simulink model "HD2_Driver_PY_v3"  (R2018a)
settings: Solver=ode1  StartTime=0.0  StopTime=inf  FixedStep=0.001  RelTol=1e-3  EnableMultiTasking=on
InitFcn:
  | % Assign block mask parameter to variable in base workspace
  | mdlPrefix_hd2_py = 'HD2_PY_';
  | mdlName_hd2_py = 'HD2_Driver_PY_v3';
  | blkName_hd2_py = 'HD2_Parameters';
  | blkRef_hd2_py = strcat(mdlName_hd2_py, '/', blkName_hd2_py);
  | 
  | % Extract list of parameters defined in the "HD2 Parameter" subsystem block
  | dialogParams_hd2_py = get_param( blkRef_hd2_py,'DialogParameters');
  | dialogParamsNames_hd2_py = fieldnames(dialogParams_hd2_py);
  | 
  | % Assign each parameter to a variable with mdlPrefix<param_name> formatted name
  | for idx = 1:numel(dialogParamsNames_hd2_py)
  |     paramVal = eval( get_param( blkRef_hd2_py, dialogParamsNames_hd2_py{idx} ) );
  |     assignin( 'base', strcat(mdlPrefix_hd2_py,dialogParamsNames_hd2_py{idx}), paramVal);
  | end
  | 
model workspace (MAT data in the model file):
  ErrTol = Simulink.Parameter
  ErrTol.Value = 0.0001
  ErrTol.DataType = 'auto'
  ErrTol.Dimensions = [1 1]
undefined symbols (not defined in the file): HD2_PY_CalibHome, HD2_PY_HandleLength, HD2_PY_HandleOffset, HD2_PY_HandleTol, HD2_PY_LinkLengths, HD2_PY_MotorAmpGains, HD2_PY_MotorAmpLimits, HD2_PY_QDirs, HD2_PY_QEnc, HD2_PY_QGains, HD2_PY_QKv, HIL, qc_get_step_size
libraries: quarc_library x30, simulink x10, simulink_extras x6
(part 1 of 2)
settings Model: SimulationMode=external  ExtModeTrigDuration=10000  Creator=glai  LastModifiedBy=mrushton
settings SolverCC: PositivePriorityOrder=on
settings RTWCC: Description=QUARC Win64 Target Using Toolchain  SystemTargetFile=quarc_win64.tlc  TemplateMakefile=quarc_default_tmf  Toolchain=QUARC win64 | nmake (64-bit Windows)  BuildConfiguration=Faster Runs
settings CodeAppCC: StateflowObjectComments=on
settings STFCustomTargetCC: TargetLangStandard=C99 (ISO)  ConcurrentExecutionCompliant=on  UseToolchainInfoCompliant=on  SystemTargetFile=quarc_win64.tlc
settings GRTTargetCC: ParMdlRefBuildCompliant=off  CompOptLevelCompliant=off  CombineOutputUpdateFcns=off  MatFileLogging=off  CPPClassGenCompliant=off  GRTInterface=on  ExtMode=on  ExtModeMexFile=quarc_comm  ExtModeMexArgs='-w -d %d -uri %u -URI_SHMEM shmem://HD2_DRIVER_PY:0','tcpip://localhost:17001'
settings ConfigComp: CovMetricSettings=dswe

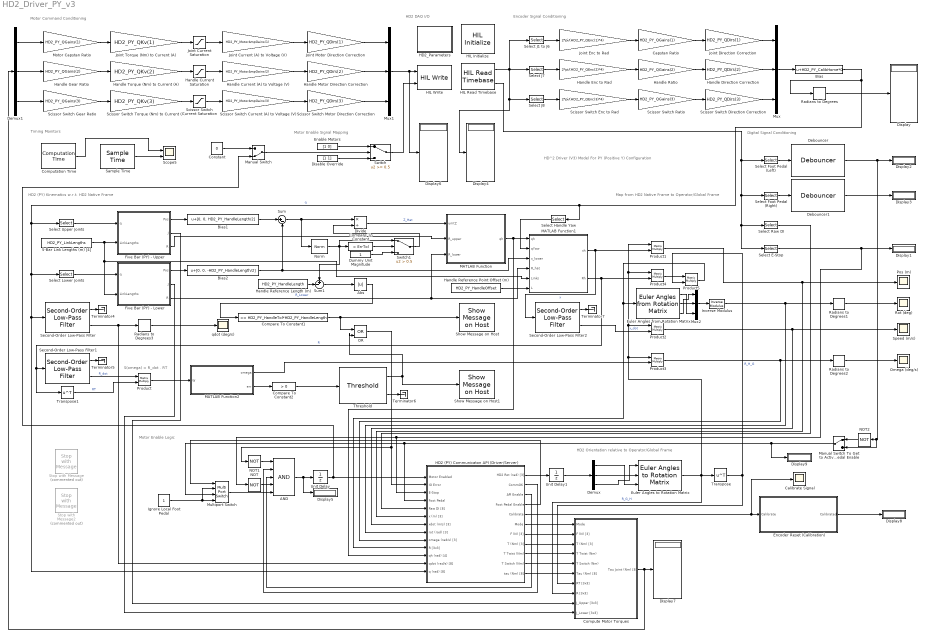
== system HD2_Driver_PY_v3 ==
  note: Motor Enable Logic
  note: Timing Monitors
  note: Map from HD2 Native Frame to Operator/Global Frame
  note: S(omega) = R_dot . RT
  note: HD2 (PY) Kinematics w.r.t. HD2 Native Frame
  note: HD2 Orientation relative to Operator/Global Frame
  note: Motor Enable Signal Mapping
  note: Motor Command Conditioning
  note: Digital Signal Conditioning
  note: Encoder Signal Conditioning
  note: HD2 DAQ I/O
  note: HD^2 Driver (V3) Model For PY (Positive Y) Configuration
  5-Bar Link Lengths (m) [4] : Constant  Value=HD2_PY_LinkLengths
  AND : Logic  Inputs=5  IconShape=distinctive  AllPortsSameDT=off  OutDataTypeStr=boolean
  Abs : Abs
  Bias : Bias  Bias=HD2_PY_CalibHome*0
  Bias1 : Bias  Bias=[0, 0, HD2_PY_HandleLength/2]
  Bias2 : Bias  Bias=[0, 0, -HD2_PY_HandleLength/2]
  Calibrate Signal : Scope
  Capstan Ratio : Gain  Gain=HD2_PY_QGains(1)
  Compare To Constant : simulink/Logic and Bit Operations/Compare To Constant  relop=>  const=ErrTol  OutDataTypeStr=boolean
  Compare To Constant1 : simulink/Logic and Bit Operations/Compare To Constant  relop=>=  const=HD2_PY_HandleTol*HD2_PY_HandleLength  OutDataTypeStr=boolean
  Compare To Constant2 : simulink/Logic and Bit Operations/Compare To Constant  relop=>  const=0  OutDataTypeStr=boolean
  Computation Time : quarc_library/Sources/Time/Computation Time  sample_time=qc_get_step_size  use_model=on  use_cpu_time=off
  Compute Motor Torques : Subsystem
  Constant : Constant  Value=0
  Debouncer : quarc_library/Discontinuities/Debouncer  init_state=Off  param_src=Specify via dialog  threshold=0.5  rise_time=0.01  fall_time=0.01
      settings: SourceProductName=QUARC Targets
  Debouncer1 : quarc_library/Discontinuities/Debouncer  init_state=Off  param_src=Specify via dialog  threshold=0.5  rise_time=0.01  fall_time=0.01
      settings: SourceProductName=QUARC Targets
  Demux : Demux  Outputs=3
  Demux1 : Demux  Outputs=[6 1 1]
  Disable Override : Constant  Value=[1 1]
  Display{,1..9} (10 alike) : Display
      settings: Decimation=100
  Divide : Product  Inputs=*/
  Dummy Unit Magnitude : Constant
  Enable Motors : Constant  Value=[1 0]
  Encoder Reset (Calibration) : Subsystem
  Euler Angles from Rotation Matrix : quarc_library/Math Operations/Matrices/Euler Angles from Rotation Matrix  menu_order=Relative Z-Y-X
      settings: SourceProductName=QUARC Targets
  Euler Angles to Rotation Matrix : quarc_library/Math Operations/Matrices/Euler Angles to Rotation Matrix  menu_order=Relative Z-Y-X
      settings: SourceProductName=QUARC Targets
  Five Bar (PY) - Lower : MATLAB Function  TreatAsAtomicUnit=on
  Five Bar (PY) - Upper : MATLAB Function  TreatAsAtomicUnit=on
  HD2 (PY) Communicaton API (Driver/Server) : Subsystem
  HD2_Parameters : Subsystem  Priority=-100  TreatAsAtomicUnit=on  mask{CalibHome=[-2, -14.5, 106, -2, -14.5, 106.5, 0, 0 ] * pi/180, HandleLength=0.175, HandleTol=0.1, HandleOffset=0.175/2, LinkLengths=[0.115, 0.28, 0.28, 0.022], QEnc=[1000, 360, 512], QGains=[1/12, 1, 1], QDirs=[-1, -1, 1], QKv=[1/115e-3, 1/0.0058, 1/0.0058], MotorAmpGains=[2.41, 2, 2], MotorAmpLimits=[5, 0.6, 0.6]}
      mask prompts: CalibHome "Joint Angles at Holder Home (rad) [8] :"; HandleLength "Handle Length/Anchor Offset (m) :"; HandleTol "Handle Length Tolerance (%) :"; HandleOffset "EE Reference Offset from base (m) :"; LinkLengths "5-Bar Link Lengths (m) [4] :"; QEnc "Encoder Resolutions (lines per rev) [3] :"; QGains "Capstan Gains/Gear Ratio [3] :"; QDirs "Direction Correction [3] :"; QKv "Torque Constant Inverse (1/Kt) (A/Nm) [3] :"; MotorAmpGains "Amplifier Resolution (V/A) [3] :"; MotorAmpLimits "Amplifier Current Limits (A) [3] :"
      mask help:
      | HD2 Parameters - PY Configuration
      |
      | The joint outputs are organized as follows (re-mapped from the encoder channel ordering):
      |
      | J1: Top 5-Bar base joint (Encoder Channel 2)
      | J2: Top 5-Bar first joint (Encoder Channel 1)
      | J3: Top 5-Bar second joint (Encoder Channel 0)
      | J4: Bottom 5-Bar base joint (Encoder Channel 5)
      | J5: Bottom 5-Bar first joint (Encoder Channel 4)
      | J6: Bottom 5-Bar second joint (Encoder Channel 3)
      | J7: Handle (Twist) joint (Encoder Channel 6)
      | J8: Scissor Switch joint (Encoder Channel 7)
      |
      | For the Joint and Motor parameters, the first 6 joints have the same values and therefore the parameter values are specified as a vector of three elements with the first element applying to J1 to J6 while the remaining elements apply to J7 and J8.
      mask init:
      | % Assign block mask parameter to variable in base workspace
      | %mdlPrefix = 'HD2_PY_';
      | 
      | %assignin( 'base', strcat(mdlPrefix,'CalibHome'), CalibHome);
      | %assignin( 'base', strcat(mdlPrefix,'HandleLength'), HandleLength);
      | %assignin( 'base', strcat(mdlPrefix,'HandleTol'), HandleTol);
      | %assignin( 'base', strcat(mdlPrefix,'HandleOffset'), HandleOffset);
      | %assignin( 'base', strcat(mdlPrefix,'LinkLengths'), LinkLengths);
      | %assignin( 'base', strcat(mdlPrefix,'QEnc'), QEnc);
      | %assignin( 'base', strcat(mdlPrefix,'QGains'), QGains);
      | %assignin( 'base', strcat(mdlPrefix,'QDirs'), QDirs);
      | %assignin( 'base', strcat(mdlPrefix,'QKv'), QKv);
      | %assignin( 'base', strcat(mdlPrefix,'MotorAmpGains'), MotorAmpGains);
      | %assignin( 'base', strcat(mdlPrefix,'MotorAmpLimits'), MotorAmpLimits);
      mask DialogControl CalibGroupVar Prompt: Calibration Parameters
      mask DialogControl ParameterGroupVar Prompt: Handle and Link Parameters
      mask DialogControl JointParamGroupVar Prompt: Joint Parameters
      mask DialogControl MotorParamGroupVar Prompt: Motor Parameters
      mask Display: disp('HD2\nParameters\n(Double-Click\nto edit)');
  HIL Initialize : quarc_library/Data Acquisition/Generic/Configuration/HIL Initialize  Priority=-99  object_name=HIL-1  board_type=qpid_e  board_number=0  board_options=enc0_dir=0;enc0_filter=1;enc0_a=1;enc0_b=1;enc0_z=0;enc0_reload=0;enc1_dir=0;enc1_filter=1;enc1_a=1;enc1_b=1;enc1_z=0;enc1_reload=0;enc2_dir=0;enc2_filter=1;enc2_a=1;enc2_b=1;enc2_z=0;enc2_reload=0;enc3_dir=0;enc3_filter=1;enc3_a=1;enc3_b=1;enc3_z=0;enc3_reload=0;enc4_dir=0;enc4_filter=1;enc4_a=1;enc4_b=1;enc4_z=0;enc4_reload=0;enc5_dir=0;enc5_filter=1;enc5_a=1;enc5_b=1;enc5_z=0;enc5_reload=0;enc6_dir=0;enc6_filter=1;enc6_a=1;enc6_b=1;enc6_z=0;enc6_reload=0;enc7_dir=0;enc7_filter=1;enc7_a=1;enc7_b=1;enc7_z=0;enc7_reload=0;ext_int_polarity=0;fuse_polarity=0;convert_polarity=0;watchdog_polarity=0;ext_int_watchdog=0;fuse_watchdog=0;trig1_watchdog=0;watchdog_to_trig1=0;watchdog_to_trig2=0;counter_to_trig0=0;trigger_adcs=0;latch_on_adc=0;pwm_immediate=0  exclusive=off  active=off  hardware_clocks=[0:16]  clock_modes=[]  initial_clock_frequencies=[]  set_clock_params_at_start=off  set_clock_params_at_switch_in=off  set_clock_frequencies_at_start=off  set_clock_frequencies_at_switch_in=off  analog_input_channels=[0:7]  analog_input_configurations=0  analog_input_maximums=10  analog_input_minimums=-10  set_analog_input_params_at_start=off  set_analog_input_params_at_switch_in=off  analog_output_channels=[0:7]  analog_output_maximums=10  analog_output_minimums=-10  initial_analog_outputs=[0]  final_analog_outputs=[0]  watchdog_analog_outputs=0  set_analog_output_params_at_start=off  set_analog_output_params_at_switch_in=off  set_analog_outputs_at_start=on  set_analog_outputs_at_switch_in=off  set_analog_outputs_at_terminate=on  set_analog_outputs_at_switch_out=off  set_analog_outputs_on_watchdog=off  digital_input_channels=[0:1,11]  digital_output_channels=[9:10]  digital_output_configuration=[]  initial_digital_outputs=[1]  final_digital_outputs=[1]  watchdog_digital_outputs=[2]  set_digital_output_params_at_start=off  set_digital_output_params_at_switch_in=off  set_digital_outputs_at_start=on  set_digital_outputs_at_switch_in=off  set_digital_outputs_at_terminate=on  set_digital_outputs_at_switch_out=off  set_digital_outputs_on_watchdog=off  encoder_channels=[0:7]  quadrature=[4]  encoder_filter_frequency=40e6/1  initial_encoder_counts=[0]  set_encoder_params_at_start=off  set_encoder_params_at_switch_in=off  set_encoder_counts_at_start=off  set_encoder_counts_at_switch_in=off  pwm_channels=[0:7]  pwm_modes=0  pwm_frequency=40e6/4096  pwm_configuration=[0]  pwm_alignment=[0]  pwm_polarity=[1]  pwm_leading_deadband=[0]  pwm_trailing_deadband=[0]  initial_pwm_outputs=[0]  final_pwm_outputs=[0]  watchdog_pwm_outputs=[0]  set_pwm_params_at_start=on  set_pwm_params_at_switch_in=off  set_pwm_outputs_at_start=on  set_pwm_outputs_at_switch_in=off  set_pwm_outputs_at_terminate=on  set_pwm_outputs_at_switch_out=off  set_pwm_outputs_on_watchdog=off  other_output_channels=[]  initial_other_outputs=[]  final_other_outputs=[]  watchdog_other_outputs=[]  set_other_outputs_at_start=off  set_other_outputs_at_switch_in=off  set_other_outputs_at_terminate=off  set_other_outputs_at_switch_out=off  set_other_outputs_on_watchdog=off
  HIL Read Timebase : quarc_library/Data Acquisition/Generic/Timebases/HIL Read Timebase  object_name=HIL-1  clock=0  analog_channels=[]  encoder_channels=[2 1 0 5 4 3 6 7]  digital_channels=[0:3, 4:7, 11]  other_channels=[]  active=on  vector_output=on  data_type_mode=Inherit via back propagation  encoder_data_type=double  digital_data_type=boolean  overflow_mode=Error on overflow  samples_in_buffer=max(ceil(1/qc_get_step_size), 1)
  HIL Write : quarc_library/Data Acquisition/Generic/Immediate I//O/HIL Write  object_name=HIL-1  analog_channels=[2 1 0 5 4 3 6 7]  pwm_channels=[]  digital_channels=[9:10]  other_channels=[]  sample_time=-1  active=on  vector_input=on
  Handle Current Saturation : Saturate  UpperLimit=HD2_PY_MotorAmpLimits(2)  LowerLimit=-HD2_PY_MotorAmpLimits(2)
  Handle Current (A) to Voltage (V) : Gain  Gain=HD2_PY_MotorAmpGains(2)
  Handle Direction Correction : Gain  Gain=HD2_PY_QDirs(2)
  Handle Enc to Rad : Gain  Gain=2*pi/(HD2_PY_QEnc(2)*4)
  Handle Gear Ratio : Gain  Gain=HD2_PY_QGains(2)
  Handle Motor Direction Correction : Gain  Gain=HD2_PY_QDirs(2)
  Handle Ratio : Gain  Gain=HD2_PY_QGains(2)
  Handle Reference Length (m) : Constant  Value=HD2_PY_HandleLength
  Handle Reference Point Offset (m) : Constant  Value=HD2_PY_HandleOffset
  Handle Torque (Nm) to Current (A) : Gain  Gain=HD2_PY_QKv(2)
  Ignore Local Foot Pedal : Constant
  Inverse Modulus : quarc_library/Discontinuities/Inverse Modulus  modulus=2*pi  output_derivative=off  output_revolutions=off  max_x=Inf  min_x=-Inf
  Joint Current (A) to Voltage (V) : Gain  Gain=HD2_PY_MotorAmpGains(1)
  Joint Current Saturation : Saturate  UpperLimit=HD2_PY_MotorAmpLimits(1)  LowerLimit=-HD2_PY_MotorAmpLimits(1)
  Joint Direction Correction : Gain  Gain=HD2_PY_QDirs(1)
  Joint Enc to Rad : Gain  Gain=2*pi/(HD2_PY_QEnc(1)*4)
  Joint Motor Direction Correction : Gain  Gain=HD2_PY_QDirs(1)
  Joint Torque (Nm) to Current (A) : Gain  Gain=HD2_PY_QKv(1)
  MATLAB Function : MATLAB Function  TreatAsAtomicUnit=on
  MATLAB Function1 : MATLAB Function  TreatAsAtomicUnit=on
  MATLAB Function2 : MATLAB Function  TreatAsAtomicUnit=on
  Manual Switch : ManualSwitch  CurrentSetting=0
  Manual Switch To Get to Active HIGH For Pedal Enable : ManualSwitch
  "Motor Capstan Ratio " : Gain  Gain=HD2_PY_QGains(1)
  Multiport Switch : MultiPortSwitch  DataPortOrder=Zero-based contiguous  Inputs=2  DataPortForDefault=Additional data port  DiagnosticForDefault=None  zeroidx=on
  Mux : Mux  Inputs=3
  Mux1 : Mux  Inputs=3
  Mux2 : Mux  Inputs=3
  NOT : Logic  Operator=NOT  IconShape=distinctive  AllPortsSameDT=off  OutDataTypeStr=boolean
  NOT1 : Logic  Operator=NOT  IconShape=distinctive  AllPortsSameDT=off  OutDataTypeStr=boolean
  NOT2 : Logic  Operator=NOT  IconShape=distinctive  AllPortsSameDT=off  OutDataTypeStr=boolean
  Norm : quarc_library/Math Operations/Vectors/Norm
      settings: SourceProductName=QUARC Targets
  OR : Logic  Operator=OR  IconShape=distinctive  AllPortsSameDT=off  OutDataTypeStr=boolean
  Omega (deg/s) : Scope
  Pos (m) : Scope
  Product{,1..5} (6 alike) : Product  Multiplication=Matrix(*)
  Radians to Degrees{,1..3} (4 alike) : simulink_extras/Transformations/Radians to Degrees
  Rot (deg) : Scope
  Sample Time : quarc_library/Sources/Time/Sample Time  Priority=-99  sample_time=qc_get_step_size
  Scissor Switch Current Saturation : Saturate  UpperLimit=HD2_PY_MotorAmpLimits(3)  LowerLimit=-HD2_PY_MotorAmpLimits(3)
  Scissor Switch Current (A) to Voltage (V) : Gain  Gain=HD2_PY_MotorAmpGains(3)
  Scissor Switch Direction Correction : Gain  Gain=HD2_PY_QDirs(3)
  Scissor Switch Enc to Rad : Gain  Gain=2*pi/(HD2_PY_QEnc(3)*4)
  Scissor Switch Gear Ratio : Gain  Gain=HD2_PY_QGains(3)
  Scissor Switch Motor Direction Correction : Gain  Gain=HD2_PY_QDirs(3)
  Scissor Switch Ratio : Gain  Gain=HD2_PY_QGains(3)
  Scissor Switch Torque (Nm) to Current (A) : Gain  Gain=HD2_PY_QKv(3)
  Scope5 : Scope  NumInputPorts=2
  Second-Order Low-Pass Filter : quarc_library/Continuous/Second-Order Low-Pass Filter  params_source=Internal (dialog parameters)  input_width=62  input_zeta=1  input_init=0
  Second-Order Low-Pass Filter1 : quarc_library/Continuous/Second-Order Low-Pass Filter  params_source=Internal (dialog parameters)  input_width=60  input_zeta=1  input_init=eye(3,3)
  Second-Order Low-Pass Filter2 : quarc_library/Continuous/Second-Order Low-Pass Filter  params_source=Internal (dialog parameters)  input_width=62  input_zeta=1  input_init=0
  Select E-Stop : Selector  InputPortWidth=9  IndexOptions=Index vector (dialog)  Indices=[9]  OutputSizes=1
  Select Foot Pedal (Left) : Selector  InputPortWidth=9  IndexOptions=Index vector (dialog)  Indices=[1]  OutputSizes=1
  Select Foot Pedal (Right) : Selector  InputPortWidth=9  IndexOptions=Index vector (dialog)  Indices=[2]  OutputSizes=1
  Select Handle Yaw : Selector  InputPortWidth=8  IndexOptions=Index vector (dialog)  Indices=[7]  OutputSizes=1
  Select J1 to J6 : Selector  InputPortWidth=8  IndexOptions=Index vector (dialog)  Indices=[1:6]  OutputSizes=1
  Select J7 : Selector  InputPortWidth=8  IndexOptions=Index vector (dialog)  Indices=[7]  OutputSizes=1
  Select J8 : Selector  InputPortWidth=8  IndexOptions=Index vector (dialog)  Indices=[8]  OutputSizes=1
  Select Lower Joints : Selector  InputPortWidth=8  IndexOptions=Index vector (dialog)  Indices=[4:6]  OutputSizes=1
  Select Raw DI : Selector  InputPortWidth=9  IndexOptions=Index vector (dialog)  Indices=[1:8]  OutputSizes=1
  Select Upper Joints : Selector  InputPortWidth=8  IndexOptions=Index vector (dialog)  Indices=[1:3]  OutputSizes=1
  Show Message on Host : quarc_library/Sinks/Error Handling/Show Message on Host  message_type=Fixed error message  message_icon=Warning  message=Inconsistent Encoder Readings (Computed Handle Length Error Exceeded Tolerance)!.
      settings: AttributesFormatString="\"%<message>\""  SourceProductName=QUARC Targets
  Show Message on Host1 : quarc_library/Sinks/Error Handling/Show Message on Host  message_type=Fixed error message  message_icon=Warning  message=Inconsistent Encoder Readings (HD2 Invalid Angular Rate)!
      settings: AttributesFormatString="\"%<message>\""  SourceProductName=QUARC Targets
  Speed (m/s) : Scope
  Stop with Message : quarc_library/Sinks/Error Handling/Stop with Message  Commented=on  message_type=Fixed error message  message_icon=Error  message=Inconsistent Encoder Readings (Computed Handle Length Error Exceeded Tolerance)!
  Stop with Message2 : quarc_library/Sinks/Error Handling/Stop with Message  Commented=on  message_type=Fixed error message  message_icon=Warning  message=Inconsistent Encoder Readings (HD2 Invalid Angular Rate)!
  Sum : Sum  Inputs=|+-
  Sum1 : Sum  Inputs=+-|
  Switch : Switch  Threshold=0.5
  Switch1 : Switch  Criteria=u2 > Threshold  Threshold=0.5
  Terminator{4..7} (4 alike) : Terminator
  Threshold : quarc_library/Discontinuities/Threshold  operator=>  param_src=Specify via dialog  threshold=0  duration=qc_get_step_size*5000
      settings: SourceProductName=QUARC Targets
  Transpose : Math  Operator=transpose  SaturateOnIntegerOverflow=on
  Transpose1 : Math  Operator=transpose  SaturateOnIntegerOverflow=on
  Unit Delay : UnitDelay  SampleTime=-1  HasFrameUpgradeWarning=on
  Unit Delay1 : UnitDelay  SampleTime=-1  HasFrameUpgradeWarning=on
  qdot (deg/s) : Scope
  wires:
  HIL Read Timebase/1 -> Select J8/1, Display4/1, Select J1 to J6/1, Select J7/1
  Select J1 to J6/1 -> Joint Enc to Rad/1
  Joint Enc to Rad/1 -> Capstan Ratio/1
  Mux/1 -> Bias/1
  Bias/1 -> Select Handle Yaw/1, Select Lower Joints/1, HD2 (PY) Communicaton API (Driver/Server)/13(q (rad) [8]), Second-Order Low-Pass Filter/1, Select Upper Joints/1, Radians to Degrees/1  "q"
  Capstan Ratio/1 -> Joint Direction Correction/1
  Joint Direction Correction/1 -> Mux/1
  Select J7/1 -> Handle Enc to Rad/1
  Handle Enc to Rad/1 -> Handle Ratio/1
  Handle Ratio/1 -> Handle Direction Correction/1
  Select J8/1 -> Scissor Switch Enc to Rad/1
  Scissor Switch Enc to Rad/1 -> Scissor Switch Ratio/1
  Scissor Switch Ratio/1 -> Scissor Switch Direction Correction/1
  Handle Direction Correction/1 -> Mux/2
  Scissor Switch Direction Correction/1 -> Mux/3
  HIL Read Timebase/2 -> Select Raw DI/1, Select E-Stop/1, Select Foot Pedal (Right)/1, Select Foot Pedal (Left)/1
  Select E-Stop/1 -> HD2 (PY) Communicaton API (Driver/Server)/3(E-Stop), NOT/1, Display1/1
  Select Foot Pedal (Right)/1 -> Debouncer1/1
  Select Foot Pedal (Left)/1 -> Debouncer/1
  Debouncer1/1 -> Display3/1
  "Motor Capstan Ratio "/1 -> Joint Torque (Nm) to Current (A)/1
  Joint Torque (Nm) to Current (A)/1 -> Joint Current Saturation/1
  Joint Current Saturation/1 -> Joint Current (A) to Voltage (V)/1
  Joint Current (A) to Voltage (V)/1 -> Joint Motor Direction Correction/1
  Mux1/1 -> Display6/1, HIL Write/1
  Joint Motor Direction Correction/1 -> Mux1/1
  Handle Current (A) to Voltage (V)/1 -> Handle Motor Direction Correction/1
  Handle Current Saturation/1 -> Handle Current (A) to Voltage (V)/1
  Handle Torque (Nm) to Current (A)/1 -> Handle Current Saturation/1
  Handle Gear Ratio/1 -> Handle Torque (Nm) to Current (A)/1
  Handle Motor Direction Correction/1 -> Mux1/2
  Scissor Switch Motor Direction Correction/1 -> Mux1/3
  Scissor Switch Gear Ratio/1 -> Scissor Switch Torque (Nm) to Current (A)/1
  Scissor Switch Torque (Nm) to Current (A)/1 -> Scissor Switch Current Saturation/1
  Scissor Switch Current Saturation/1 -> Scissor Switch Current (A) to Voltage (V)/1
  Scissor Switch Current (A) to Voltage (V)/1 -> Scissor Switch Motor Direction Correction/1
  Enable Motors/1 -> Switch/1
  Unit Delay/1 -> HD2 (PY) Communicaton API (Driver/Server)/1(Motor Enabled), Manual Switch/2
  Disable Override/1 -> Switch/3
  Switch/1 -> HIL Write/2
  Demux/2 -> Euler Angles to Rotation Matrix/2
  Demux/1 -> Euler Angles to Rotation Matrix/3
  Demux/3 -> Euler Angles to Rotation Matrix/1
  Euler Angles to Rotation Matrix/1 -> Transpose/1, Compute Motor Torques/8(R [3x3]), Product1/1, Product4/1, Product2/1, Product3/1  "R_G_H"
  5-Bar Link Lengths (m) [4]/1 -> MATLAB Function1/5(Links), Five Bar (PY) - Lower/2(LinkLengths), Five Bar (PY) - Upper/2(LinkLengths)
  Five Bar (PY) - Upper/1(Pos) -> Bias1/1
  Five Bar (PY) - Lower/1(Pos) -> Bias2/1
  Bias1/1 -> Sum/1
  Bias2/1 -> MATLAB Function1/3(x_lower), Sum/2
  Sum/1 -> Divide/1, Norm/1
  Norm/1 -> Sum1/1, Switch1/1, Compare To Constant/1
  Compare To Constant/1 -> Switch1/2
  Dummy Unit Magnitude/1 -> Switch1/3
  Switch1/1 -> Divide/2
  Divide/1 -> MATLAB Function/1(unitZ)  "Z_Hat"
  Five Bar (PY) - Lower/3(R) -> MATLAB Function1/4(R_hat), MATLAB Function/3(R_lower)  "R_Lower"
  MATLAB Function/1(qh) -> MATLAB Function1/1(qh), HD2 (PY) Communicaton API (Driver/Server)/11(qh (rad) [4])
  Handle Reference Point Offset (m)/1 -> MATLAB Function1/6(L)
  Select Handle Yaw/1 -> MATLAB Function1/2(qYaw)
  Five Bar (PY) - Upper/2(J) -> Compute Motor Torques/9(J_Upper [3x3])
  Five Bar (PY) - Lower/2(J) -> Compute Motor Torques/10(J_Lower [3x3])
  Select Upper Joints/1 -> Five Bar (PY) - Upper/1(q)
  Five Bar (PY) - Upper/3(R) -> MATLAB Function/2(R_upper)
  Select Lower Joints/1 -> Five Bar (PY) - Lower/1(q)
  Handle Reference Length (m)/1 -> Sum1/2
  Sum1/1 -> Abs/1
  Abs/1 -> Compare To Constant1/1
  Compare To Constant1/1 -> Show Message on Host/1, OR/1
  Second-Order Low-Pass Filter/1 -> Terminator4/1
  MATLAB Function1/2(Rh) -> Product4/2, Transpose1/1, Second-Order Low-Pass Filter1/1  "R"
  Second-Order Low-Pass Filter1/2 -> Product/1  "R_dot"
  Transpose1/1 -> Product/2  "RT"
  Second-Order Low-Pass Filter1/1 -> Terminator5/1
  Product/1 -> MATLAB Function2/1(W)
  MATLAB Function2/2(err) -> Compare To Constant2/1
  Compare To Constant2/1 -> Threshold/1
  Threshold/1 -> Show Message on Host1/1, OR/2
  Threshold/2 -> Terminator6/1
  MATLAB Function1/1(xh) -> Second-Order Low-Pass Filter2/1, Product1/2  "x"
  Second-Order Low-Pass Filter2/1 -> Terminator7/1
  Second-Order Low-Pass Filter2/2 -> Product2/2  "x_dot"
  MATLAB Function2/1(omega) -> Product3/2
  Product4/1 -> Product5/1
  Transpose/1 -> Product5/2, Compute Motor Torques/7(RT [3x3])  "R_H_G"
  Product5/1 -> HD2 (PY) Communicaton API (Driver/Server)/10(R [3x3]), Euler Angles from Rotation Matrix/1
  Euler Angles from Rotation Matrix/2 -> Mux2/2
  Euler Angles from Rotation Matrix/1 -> Mux2/3
  Euler Angles from Rotation Matrix/3 -> Mux2/1
  Mux2/1 -> Inverse Modulus/1
  Product1/1 -> HD2 (PY) Communicaton API (Driver/Server)/6(x (m) [3]), Pos (m)/1
  Inverse Modulus/1 -> Radians to Degrees1/1, HD2 (PY) Communicaton API (Driver/Server)/8(rot (rad) [3])
  Product2/1 -> Speed (m/s)/1, HD2 (PY) Communicaton API (Driver/Server)/7(xdot (m/s) [3])
  Product3/1 -> HD2 (PY) Communicaton API (Driver/Server)/9(omega (rad/s) [3]), Radians to Degrees2/1
  Second-Order Low-Pass Filter/2 -> Radians to Degrees3/1, HD2 (PY) Communicaton API (Driver/Server)/12(qdot (rad/s) [8])
  Radians to Degrees/1 -> Display/1
  Computation Time/1 -> Scope5/1
  Sample Time/1 -> Scope5/2
  OR/1 -> HD2 (PY) Communicaton API (Driver/Server)/2(IO Error), NOT1/1
  HD2 (PY) Communicaton API (Driver/Server)/1(HD2 Rot (rad) [3]) -> Unit Delay1/1
  Select Raw DI/1 -> HD2 (PY) Communicaton API (Driver/Server)/5(Raw DI [8])
  AND/1 -> Display5/1, Unit Delay/1
  HD2 (PY) Communicaton API (Driver/Server)/4(Foot Pedal Enable) -> Multiport Switch/1
  Ignore Local Foot Pedal/1 -> Multiport Switch/2, Multiport Switch/4
  HD2 (PY) Communicaton API (Driver/Server)/7(F (N) [3]) -> Compute Motor Torques/2(F (N) [3])
  HD2 (PY) Communicaton API (Driver/Server)/8(T (Nm) [3]) -> Compute Motor Torques/3(T (Nm) [3])
  HD2 (PY) Communicaton API (Driver/Server)/9(T Twist (Nm)) -> Compute Motor Torques/4(T Twist (Nm))
  HD2 (PY) Communicaton API (Driver/Server)/10(T Switch (Nm)) -> Compute Motor Torques/5(T Switch (Nm))
  HD2 (PY) Communicaton API (Driver/Server)/11(tau (Nm) [8]) -> Compute Motor Torques/6(Tau (Nm) [8])
  HD2 (PY) Communicaton API (Driver/Server)/6(Mode) -> Compute Motor Torques/1(Mode)
  Demux1/1 -> "Motor Capstan Ratio "/1
  Demux1/2 -> Handle Gear Ratio/1
  Demux1/3 -> Scissor Switch Gear Ratio/1
  Unit Delay1/1 -> Demux/1
  Constant/1 -> Manual Switch/1
  Manual Switch/1 -> Switch/2
  Radians to Degrees1/1 -> Rot (deg)/1
  Radians to Degrees2/1 -> Omega (deg/s)/1
  Compute Motor Torques/1(Tau Joint (Nm) [8]) -> Demux1/1, Display7/1
  Multiport Switch/1 -> AND/5
  NOT/1 -> AND/4
  NOT1/1 -> AND/1
  HD2 (PY) Communicaton API (Driver/Server)/2(CommOK) -> AND/2
  HD2 (PY) Communicaton API (Driver/Server)/3(API Enable) -> AND/3
  HD2 (PY) Communicaton API (Driver/Server)/5(Calibrate) -> Calibrate Signal/1, Encoder Reset (Calibration)/1(Calibrate)
  Encoder Reset (Calibration)/1(Calibrated) -> Display8/1
  NOT2/1 -> Manual Switch To Get to Active HIGH For Pedal Enable/1
  Debouncer/1 -> Manual Switch To Get to Active HIGH For Pedal Enable/2, NOT2/1, Display2/1
  Manual Switch To Get to Active HIGH For Pedal Enable/1 -> Display9/1, HD2 (PY) Communicaton API (Driver/Server)/4(Foot Pedal), Multiport Switch/3
  Radians to Degrees3/1 -> qdot (deg/s)/1

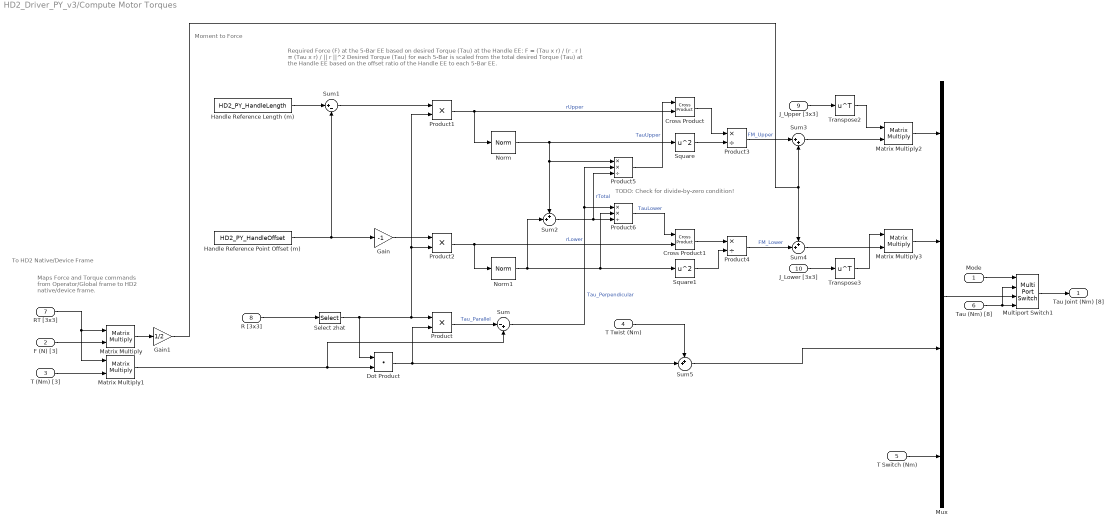
== system HD2_Driver_PY_v3/Compute Motor Torques ==
  note: Moment to Force
  note: To HD2 Native/Device Frame
  note: Maps Force and Torque commands
      | from Operator/Global frame
      | to HD2 native/device frame.
  note: TODO: Check for divide-by-zero condition!
  note: Required Force (F) at the 5-Bar EE based on desired Torque (Tau) at the Handle EE:
      |
      | F = (Tau x r) / (r . r ) = (Tau x r) / || r ||^2
      |
      | Desired Torque (Tau) for each 5-Bar is scaled from the total desired Torque (Tau) at the Handle EE based on the offset ratio of the Handle EE to each 5-Bar EE.
  Mode : Inport
  F (N) [3] : Inport  Port=2
  T (Nm) [3] : Inport  Port=3
  T Twist (Nm) : Inport  Port=4
  T Switch (Nm) : Inport  Port=5
  Tau (Nm) [8] : Inport  Port=6
  RT [3x3] : Inport  Port=7
  R [3x3] : Inport  Port=8
  J_Upper [3x3] : Inport  Port=9
  J_Lower [3x3] : Inport  Port=10
  Cross Product : quarc_library/Math Operations/Vectors/Cross Product
      settings: SourceProductName=QUARC Targets
  Cross Product1 : quarc_library/Math Operations/Vectors/Cross Product
      settings: SourceProductName=QUARC Targets
  Dot Product : DotProduct  InputSameDT=on  OutDataTypeStr=Inherit: Inherit via internal rule
  Gain : Gain  Gain=-1
  Gain1 : Gain  Gain=1/2
  Handle Reference Length (m) : Constant  Value=HD2_PY_HandleLength
  Handle Reference Point Offset (m) : Constant  Value=HD2_PY_HandleOffset
  Matrix Multiply{,1..3} (4 alike) : Product  Multiplication=Matrix(*)
  Multiport Switch1 : MultiPortSwitch  DataPortOrder=Zero-based contiguous  DiagnosticForDefault=None  zeroidx=on
  Mux : Mux
  Norm : quarc_library/Math Operations/Vectors/Norm
      settings: SourceProductName=QUARC Targets
  Norm1 : quarc_library/Math Operations/Vectors/Norm
      settings: SourceProductName=QUARC Targets
  Product : Product
  Product1 : Product
  Product2 : Product
  Product3 : Product  Inputs=*/
  Product4 : Product  Inputs=*/
  Product5 : Product  Inputs=**/
  Product6 : Product  Inputs=**/
  Select zhat : Selector  NumberOfDimensions=2  InputPortWidth=3  IndexOptions=Index vector (dialog),Index vector (dialog)  Indices=[1:3],3  OutputSizes=1,1
  Square : Math  Operator=square  SaturateOnIntegerOverflow=on
  Square1 : Math  Operator=square  SaturateOnIntegerOverflow=on
  Sum : Sum  Inputs=|-+
  Sum1 : Sum  Inputs=|+-
  Sum2 : Sum  Inputs=++|
  Sum3 : Sum  Inputs=|++
  Sum4 : Sum  Inputs=++|
  Sum5 : Sum  Inputs=++|
  Transpose2 : Math  Operator=transpose  SaturateOnIntegerOverflow=on
  Transpose3 : Math  Operator=transpose  SaturateOnIntegerOverflow=on
  Tau Joint (Nm) [8] : Outport  VectorParamsAs1DForOutWhenUnconnected=off
  wires:
  RT [3x3]/1 -> Matrix Multiply1/1, Matrix Multiply/1
  F (N) [3]/1 -> Matrix Multiply/2
  T (Nm) [3]/1 -> Matrix Multiply1/2
  Square/1 -> Product3/2
  Cross Product/1 -> Product3/1
  Handle Reference Point Offset (m)/1 -> Gain/1, Sum1/2
  Handle Reference Length (m)/1 -> Sum1/1
  Product6/1 -> Cross Product1/1  "TauLower"
  Cross Product1/1 -> Product4/1
  Sum1/1 -> Product1/1
  Sum2/1 -> Product5/3, Product6/3  "rTotal"
  Product3/1 -> Sum3/1  "FM_Upper"
  Dot Product/1 -> Sum5/2, Product/2
  Norm1/1 -> Sum2/2, Product6/2, Square1/1
  Select zhat/1 -> Product1/2, Product2/2, Product/1, Dot Product/1
  Norm/1 -> Product5/1, Sum2/1, Square/1
  Square1/1 -> Product4/2
  Product/1 -> Sum/1  "Tau_Parallel"
  Product5/1 -> Cross Product/1  "TauUpper"
  Gain/1 -> Product2/1
  Product2/1 -> Norm1/1, Cross Product1/2  "rLower"
  Product1/1 -> Norm/1, Cross Product/2  "rUpper"
  R [3x3]/1 -> Select zhat/1
  Matrix Multiply1/1 -> Sum/2, Dot Product/2
  Sum/1 -> Product6/1, Product5/2  "Tau_Perpendicular"
  Matrix Multiply/1 -> Gain1/1
  Product4/1 -> Sum4/2  "FM_Lower"
  Gain1/1 -> Sum3/2, Sum4/1
  Sum3/1 -> Matrix Multiply2/2
  J_Upper [3x3]/1 -> Transpose2/1
  Transpose2/1 -> Matrix Multiply2/1
  Sum4/1 -> Matrix Multiply3/2
  J_Lower [3x3]/1 -> Transpose3/1
  Transpose3/1 -> Matrix Multiply3/1
  T Twist (Nm)/1 -> Sum5/1
  Matrix Multiply3/1 -> Mux/2
  Matrix Multiply2/1 -> Mux/1
  Mode/1 -> Multiport Switch1/1
  Mux/1 -> Multiport Switch1/3
  Multiport Switch1/1 -> Tau Joint (Nm) [8]/1
  Tau (Nm) [8]/1 -> Multiport Switch1/2, Multiport Switch1/4
  T Switch (Nm)/1 -> Mux/4
  Sum5/1 -> Mux/3

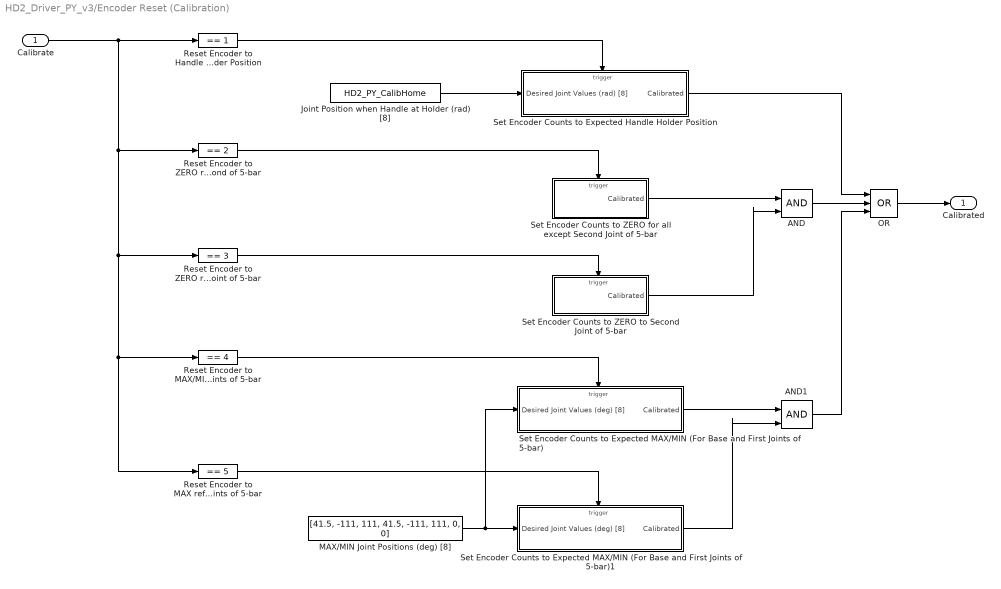
== system HD2_Driver_PY_v3/Encoder Reset (Calibration) ==
  Calibrate : Inport
  AND : Logic  IconShape=distinctive  AllPortsSameDT=off  OutDataTypeStr=boolean
  AND1 : Logic  IconShape=distinctive  AllPortsSameDT=off  OutDataTypeStr=boolean
  Joint Position when Handle at Holder (rad) [8] : Constant  Value=HD2_PY_CalibHome
  MAX/MIN Joint Positions (deg) [8] : Constant  Value=[41.5, -111, 111, 41.5, -111, 111, 0, 0]
  OR : Logic  Operator=OR  Inputs=3  IconShape=distinctive  AllPortsSameDT=off  OutDataTypeStr=boolean
  Reset Encoder to Handle Holder Position : simulink/Logic and Bit Operations/Compare To Constant  relop===  const=1  OutDataTypeStr=boolean
  Reset Encoder to MAX reference position For Second joints of 5-bar : simulink/Logic and Bit Operations/Compare To Constant  relop===  const=5  OutDataTypeStr=boolean
  Reset Encoder to MAX/MIN reference position For Base and First joints of 5-bar : simulink/Logic and Bit Operations/Compare To Constant  relop===  const=4  OutDataTypeStr=boolean
  Reset Encoder to ZERO reference position For ALL joints except Second of 5-bar : simulink/Logic and Bit Operations/Compare To Constant  relop===  const=2  OutDataTypeStr=boolean
  Reset Encoder to ZERO reference position For Second Joint of 5-bar : simulink/Logic and Bit Operations/Compare To Constant  relop===  const=3  OutDataTypeStr=boolean
  Set Encoder Counts to Expected Handle Holder Position : Subsystem  TreatAsAtomicUnit=on
  Set Encoder Counts to Expected MAX/MIN (For Base and First Joints of 5-bar) : Subsystem  TreatAsAtomicUnit=on
  Set Encoder Counts to Expected MAX/MIN (For Base and First Joints of 5-bar)1 : Subsystem  TreatAsAtomicUnit=on
  Set Encoder Counts to ZERO for all except Second Joint of 5-bar : Subsystem  TreatAsAtomicUnit=on
  Set Encoder Counts to ZERO to Second Joint of 5-bar : Subsystem  TreatAsAtomicUnit=on
  Calibrated : Outport  VectorParamsAs1DForOutWhenUnconnected=off
  wires:
  Calibrate/1 -> Reset Encoder to ZERO reference position For ALL joints except Second of 5-bar/1, Reset Encoder to MAX reference position For Second joints of 5-bar/1, Reset Encoder to MAX/MIN reference position For Base and First joints of 5-bar/1, Reset Encoder to ZERO reference position For Second Joint of 5-bar/1, Reset Encoder to Handle Holder Position/1
  Reset Encoder to Handle Holder Position/1 -> Set Encoder Counts to Expected Handle Holder Position/Trigger
  Joint Position when Handle at Holder (rad) [8]/1 -> Set Encoder Counts to Expected Handle Holder Position/1(Desired Joint Values (rad) [8])
  Reset Encoder to ZERO reference position For ALL joints except Second of 5-bar/1 -> Set Encoder Counts to ZERO for all except Second Joint of 5-bar/Trigger
  Reset Encoder to ZERO reference position For Second Joint of 5-bar/1 -> Set Encoder Counts to ZERO to Second Joint of 5-bar/Trigger
  Set Encoder Counts to ZERO for all except Second Joint of 5-bar/1(Calibrated) -> AND/1
  Set Encoder Counts to ZERO to Second Joint of 5-bar/1(Calibrated) -> AND/2
  AND/1 -> OR/2
  Set Encoder Counts to Expected Handle Holder Position/1(Calibrated) -> OR/1
  OR/1 -> Calibrated/1
  Reset Encoder to MAX/MIN reference position For Base and First joints of 5-bar/1 -> Set Encoder Counts to Expected MAX/MIN (For Base and First Joints of 5-bar)/Trigger
  MAX/MIN Joint Positions (deg) [8]/1 -> Set Encoder Counts to Expected MAX/MIN (For Base and First Joints of 5-bar)/1(Desired Joint Values (deg) [8]), Set Encoder Counts to Expected MAX/MIN (For Base and First Joints of 5-bar)1/1(Desired Joint Values (deg) [8])
  Set Encoder Counts to Expected MAX/MIN (For Base and First Joints of 5-bar)/1(Calibrated) -> AND1/1
  Reset Encoder to MAX reference position For Second joints of 5-bar/1 -> Set Encoder Counts to Expected MAX/MIN (For Base and First Joints of 5-bar)1/Trigger
  Set Encoder Counts to Expected MAX/MIN (For Base and First Joints of 5-bar)1/1(Calibrated) -> AND1/2
  AND1/1 -> OR/3

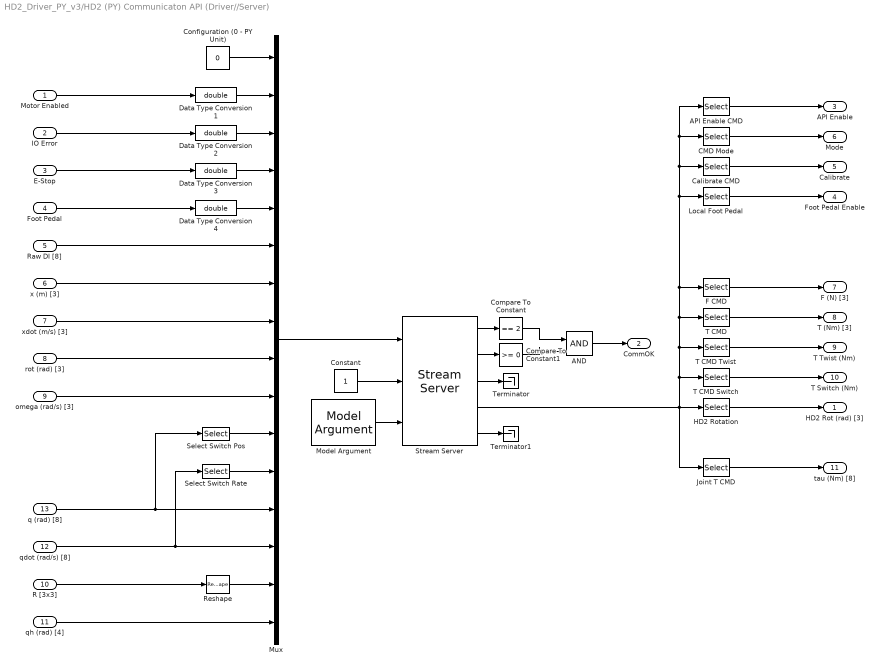
== system HD2_Driver_PY_v3/HD2 (PY) Communicaton API (Driver//Server) ==
  Motor Enabled : Inport
  IO Error : Inport  Port=2
  E-Stop : Inport  Port=3
  Foot Pedal : Inport  Port=4
  Raw DI [8] : Inport  Port=5
  x (m) [3] : Inport  Port=6
  xdot (m/s) [3] : Inport  Port=7
  rot (rad) [3] : Inport  Port=8
  omega (rad/s) [3] : Inport  Port=9
  R [3x3] : Inport  Port=10
  qh (rad) [4] : Inport  Port=11
  qdot (rad/s) [8] : Inport  Port=12
  q (rad) [8] : Inport  Port=13
  AND : Logic  IconShape=distinctive  AllPortsSameDT=off  OutDataTypeStr=boolean
  API Enable CMD : Selector  InputPortWidth=23  IndexOptions=Index vector (dialog)  Indices=[1]  OutputSizes=1
  CMD Mode : Selector  InputPortWidth=23  IndexOptions=Index vector (dialog)  Indices=[2]  OutputSizes=1
  Calibrate CMD : Selector  InputPortWidth=23  IndexOptions=Index vector (dialog)  Indices=[3]  OutputSizes=1
  Compare To Constant : simulink/Logic and Bit Operations/Compare To Constant  relop===  const=2  OutDataTypeStr=boolean
  Compare To Constant1 : simulink/Logic and Bit Operations/Compare To Constant  relop=>=  const=0  OutDataTypeStr=boolean
  Configuration (0 - PY Unit) : Constant  Value=0
  Constant : Constant
  Data Type Conversion{1..4} (4 alike) : DataTypeConversion  OutDataTypeStr=double
  F CMD : Selector  InputPortWidth=23  IndexOptions=Index vector (dialog)  Indices=[5:7]  OutputSizes=1
  HD2 Rotation : Selector  InputPortWidth=23  IndexOptions=Index vector (dialog)  Indices=[13:15]  OutputSizes=1
  Joint T CMD : Selector  InputPortWidth=23  IndexOptions=Index vector (dialog)  Indices=[16:23]  OutputSizes=1
  Local Foot Pedal : Selector  InputPortWidth=23  IndexOptions=Index vector (dialog)  Indices=[4]  OutputSizes=1
  Model Argument : quarc_library/Sources/Signals/Model Argument  argument_name=URI_SHMEM  has_value=on  data_type_mode=Specify via dialog  data_type=char  max_length=80  default_value=0  variable_size=off
      settings: AttributesFormatString=(-%<argument_name>)  SourceProductName=QUARC Targets
  Mux : Mux  Inputs=[1 1 1 1 1 8 3 3 3 3 1 1 8 8 9 4]
  Reshape : Reshape
  Select Switch Pos : Selector  InputPortWidth=8  IndexOptions=Index vector (dialog)  Indices=[8]  OutputSizes=1
  Select Switch Rate : Selector  InputPortWidth=8  IndexOptions=Index vector (dialog)  Indices=[8]  OutputSizes=1
  Stream Server : quarc_library/Communications/Basic/Stream Server  uri_source=External input port  uri=tcpip://remotehost:18000  send_buffer_size=2048  receive_buffer_size=2048  byte_order=little endian (Intel - LSB first)  optimization=Minimum latency  send_options=Send most recent data  receive_options=Receive most recent data  default_value=zeros(1,23)  sample_time=qc_get_step_size  active=off  implementation=Use blocking I/O in a separate thread  send_fifo_size=1000  receive_fifo_size=1000  send_priority=0  receive_priority=0  send_dimensions=off  receive_dimensions=off  max_dimensions=-1  data_type=double  type_expr=BusObject
  T CMD : Selector  InputPortWidth=23  IndexOptions=Index vector (dialog)  Indices=[8:10]  OutputSizes=1
  T CMD Switch : Selector  InputPortWidth=23  IndexOptions=Index vector (dialog)  Indices=[12]  OutputSizes=1
  T CMD Twist : Selector  InputPortWidth=23  IndexOptions=Index vector (dialog)  Indices=[11]  OutputSizes=1
  Terminator : Terminator
  Terminator1 : Terminator
  HD2 Rot (rad) [3] : Outport  VectorParamsAs1DForOutWhenUnconnected=off
  CommOK : Outport  Port=2  VectorParamsAs1DForOutWhenUnconnected=off
  API Enable : Outport  Port=3  VectorParamsAs1DForOutWhenUnconnected=off
  Foot Pedal Enable : Outport  Port=4  VectorParamsAs1DForOutWhenUnconnected=off
  Calibrate : Outport  Port=5  VectorParamsAs1DForOutWhenUnconnected=off
  Mode : Outport  Port=6  VectorParamsAs1DForOutWhenUnconnected=off
  F (N) [3] : Outport  Port=7  VectorParamsAs1DForOutWhenUnconnected=off
  T (Nm) [3] : Outport  Port=8  VectorParamsAs1DForOutWhenUnconnected=off
  T Twist (Nm) : Outport  Port=9  VectorParamsAs1DForOutWhenUnconnected=off
  T Switch (Nm) : Outport  Port=10  VectorParamsAs1DForOutWhenUnconnected=off
  tau (Nm) [8] : Outport  Port=11  VectorParamsAs1DForOutWhenUnconnected=off
  wires:
  Compare To Constant/1 -> AND/1
  Compare To Constant1/1 -> AND/2
  Stream Server/1 -> Compare To Constant/1
  Stream Server/2 -> Compare To Constant1/1
  Stream Server/3 -> Terminator/1
  Model Argument/1 -> Stream Server/3
  Constant/1 -> Stream Server/2
  Stream Server/5 -> Terminator1/1
  AND/1 -> CommOK/1
  Configuration (0 - PY Unit)/1 -> Mux/1
  Motor Enabled/1 -> Data Type Conversion1/1
  IO Error/1 -> Data Type Conversion2/1
  E-Stop/1 -> Data Type Conversion3/1
  Foot Pedal/1 -> Data Type Conversion4/1
  Raw DI [8]/1 -> Mux/6
  x (m) [3]/1 -> Mux/7
  xdot (m/s) [3]/1 -> Mux/8
  rot (rad) [3]/1 -> Mux/9
  omega (rad/s) [3]/1 -> Mux/10
  q (rad) [8]/1 -> Mux/13, Select Switch Pos/1
  qdot (rad/s) [8]/1 -> Mux/14, Select Switch Rate/1
  R [3x3]/1 -> Reshape/1
  Reshape/1 -> Mux/15
  Stream Server/4 -> Calibrate CMD/1, CMD Mode/1, API Enable CMD/1, Local Foot Pedal/1, F CMD/1, T CMD/1, T CMD Twist/1, T CMD Switch/1, HD2 Rotation/1, Joint T CMD/1
  API Enable CMD/1 -> API Enable/1
  CMD Mode/1 -> Mode/1
  Local Foot Pedal/1 -> Foot Pedal Enable/1
  F CMD/1 -> F (N) [3]/1
  T CMD/1 -> T (Nm) [3]/1
  T CMD Twist/1 -> T Twist (Nm)/1
  T CMD Switch/1 -> T Switch (Nm)/1
  HD2 Rotation/1 -> HD2 Rot (rad) [3]/1
  Joint T CMD/1 -> tau (Nm) [8]/1
  Mux/1 -> Stream Server/1
  Data Type Conversion1/1 -> Mux/2
  Data Type Conversion2/1 -> Mux/3
  Data Type Conversion3/1 -> Mux/4
  Data Type Conversion4/1 -> Mux/5
  Select Switch Pos/1 -> Mux/11
  Select Switch Rate/1 -> Mux/12
  qh (rad) [4]/1 -> Mux/16
  Calibrate CMD/1 -> Calibrate/1

== system HD2_Driver_PY_v3/HD2_Parameters ==
  note: Parameters defined in the mask of this subsystem is read by the code defined in the InitFcn Callback function of the model.
      |
      | These values are then assigned to a corresponding variable in the base workspace.
  note: This is an atomic subsystem

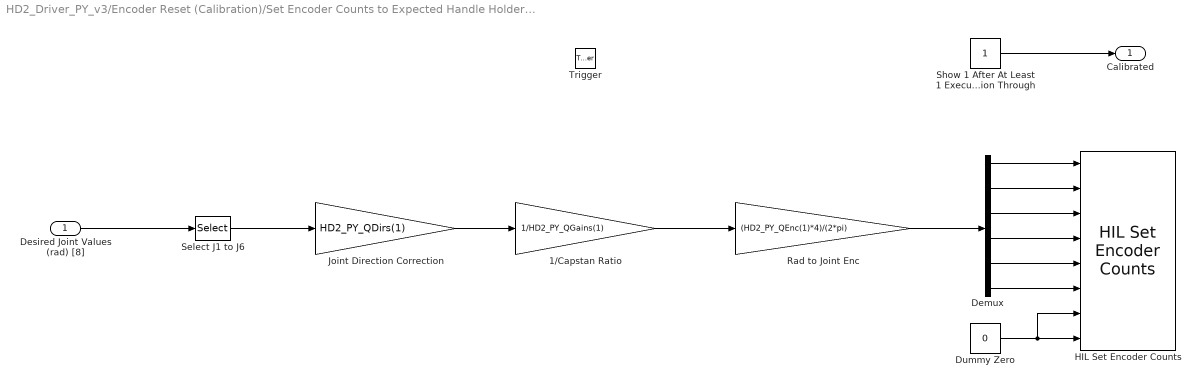
== system HD2_Driver_PY_v3/Encoder Reset (Calibration)/Set Encoder Counts to Expected Handle Holder Position ==
  Desired Joint Values (rad) [8] : Inport
  Trigger : TriggerPort  VariantControl=Variant
  1/Capstan Ratio : Gain  Gain=1/HD2_PY_QGains(1)
  Demux : Demux  Outputs=6
  Dummy Zero : Constant  Value=0
  HIL Set Encoder Counts : quarc_library/Data Acquisition/Generic/Configuration/HIL Set Encoder Counts  object_name=HIL-1  channels=[2 1 0 5 4 3 6 7]  source=external  counts=0  sample_time=-1  active=on  vector_input=off
      settings: AttributesFormatString=(%<object_name>)  SourceProductName=QUARC Targets
  Joint Direction Correction : Gain  Gain=HD2_PY_QDirs(1)
  Rad to Joint Enc : Gain  Gain=(HD2_PY_QEnc(1)*4)/(2*pi)
  Select J1 to J6 : Selector  InputPortWidth=8  IndexOptions=Index vector (dialog)  Indices=[1:6]  OutputSizes=1
  Show 1 After At Least 1 Execution Through : Constant
  Calibrated : Outport  InitialOutput=[0]  VectorParamsAs1DForOutWhenUnconnected=off
  wires:
  1/Capstan Ratio/1 -> Rad to Joint Enc/1
  Dummy Zero/1 -> HIL Set Encoder Counts/7, HIL Set Encoder Counts/8
  Desired Joint Values (rad) [8]/1 -> Select J1 to J6/1
  Rad to Joint Enc/1 -> Demux/1
  Show 1 After At Least 1 Execution Through/1 -> Calibrated/1
  Demux/4 -> HIL Set Encoder Counts/4
  Demux/1 -> HIL Set Encoder Counts/1
  Demux/3 -> HIL Set Encoder Counts/3
  Demux/2 -> HIL Set Encoder Counts/2
  Demux/5 -> HIL Set Encoder Counts/5
  Demux/6 -> HIL Set Encoder Counts/6
  Joint Direction Correction/1 -> 1/Capstan Ratio/1
  Select J1 to J6/1 -> Joint Direction Correction/1

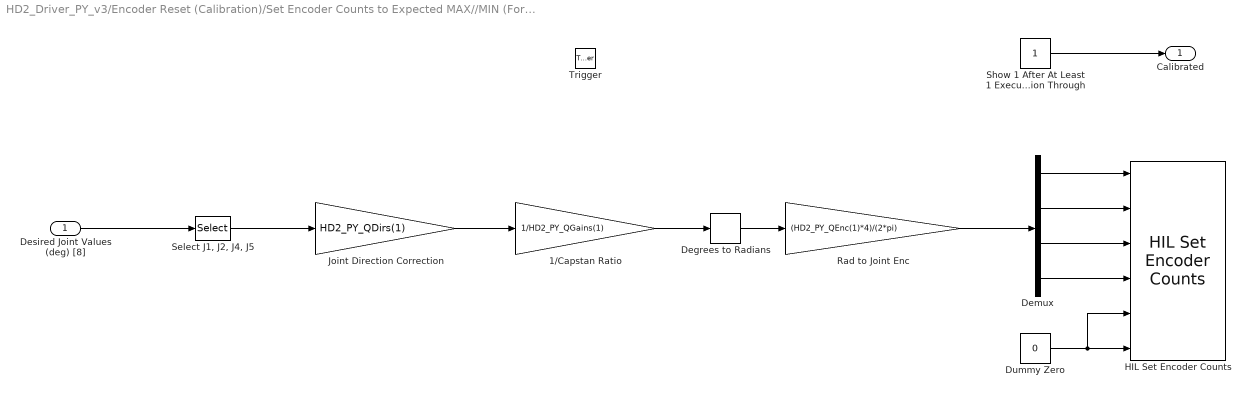
== system HD2_Driver_PY_v3/Encoder Reset (Calibration)/Set Encoder Counts to Expected MAX//MIN (For Base and First Joints of 5-bar) ==
  Desired Joint Values (deg) [8] : Inport
  Trigger : TriggerPort  VariantControl=Variant
  1/Capstan Ratio : Gain  Gain=1/HD2_PY_QGains(1)
  Degrees to Radians : simulink_extras/Transformations/Degrees to Radians
  Demux : Demux
  Dummy Zero : Constant  Value=0
  HIL Set Encoder Counts : quarc_library/Data Acquisition/Generic/Configuration/HIL Set Encoder Counts  object_name=HIL-1  channels=[2 1 5 4 6 7]  source=external  counts=0  sample_time=-1  active=on  vector_input=off
      settings: AttributesFormatString=(%<object_name>)  SourceProductName=QUARC Targets
  Joint Direction Correction : Gain  Gain=HD2_PY_QDirs(1)
  Rad to Joint Enc : Gain  Gain=(HD2_PY_QEnc(1)*4)/(2*pi)
  "Select J1, J2, J4, J5" : Selector  InputPortWidth=8  IndexOptions=Index vector (dialog)  Indices=[1,2,4,5]  OutputSizes=1
  Show 1 After At Least 1 Execution Through : Constant
  Calibrated : Outport  InitialOutput=[0]  VectorParamsAs1DForOutWhenUnconnected=off
  wires:
  "Select J1, J2, J4, J5"/1 -> Joint Direction Correction/1
  Joint Direction Correction/1 -> 1/Capstan Ratio/1
  Demux/2 -> HIL Set Encoder Counts/2
  Demux/3 -> HIL Set Encoder Counts/3
  Demux/1 -> HIL Set Encoder Counts/1
  Demux/4 -> HIL Set Encoder Counts/4
  Show 1 After At Least 1 Execution Through/1 -> Calibrated/1
  Rad to Joint Enc/1 -> Demux/1
  Desired Joint Values (deg) [8]/1 -> "Select J1, J2, J4, J5"/1
  Dummy Zero/1 -> HIL Set Encoder Counts/5, HIL Set Encoder Counts/6
  1/Capstan Ratio/1 -> Degrees to Radians/1
  Degrees to Radians/1 -> Rad to Joint Enc/1

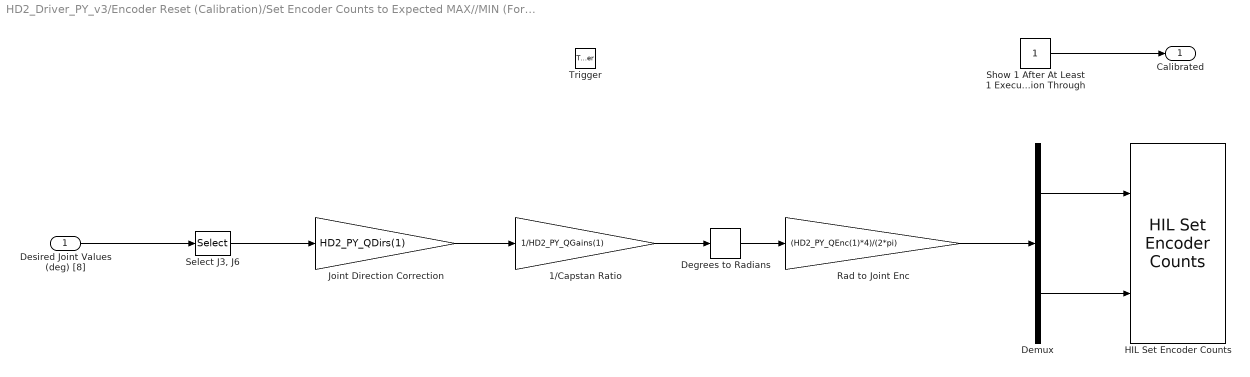
== system HD2_Driver_PY_v3/Encoder Reset (Calibration)/Set Encoder Counts to Expected MAX//MIN (For Base and First Joints of 5-bar)1 ==
  Desired Joint Values (deg) [8] : Inport
  Trigger : TriggerPort  VariantControl=Variant
  1/Capstan Ratio : Gain  Gain=1/HD2_PY_QGains(1)
  Degrees to Radians : simulink_extras/Transformations/Degrees to Radians
  Demux : Demux  Outputs=2
  HIL Set Encoder Counts : quarc_library/Data Acquisition/Generic/Configuration/HIL Set Encoder Counts  object_name=HIL-1  channels=[0 3]  source=external  counts=0  sample_time=-1  active=on  vector_input=off
      settings: AttributesFormatString=(%<object_name>)  SourceProductName=QUARC Targets
  Joint Direction Correction : Gain  Gain=HD2_PY_QDirs(1)
  Rad to Joint Enc : Gain  Gain=(HD2_PY_QEnc(1)*4)/(2*pi)
  "Select J3, J6" : Selector  InputPortWidth=8  IndexOptions=Index vector (dialog)  Indices=[3,6]  OutputSizes=1
  Show 1 After At Least 1 Execution Through : Constant
  Calibrated : Outport  InitialOutput=[0]  VectorParamsAs1DForOutWhenUnconnected=off
  wires:
  Degrees to Radians/1 -> Rad to Joint Enc/1
  1/Capstan Ratio/1 -> Degrees to Radians/1
  Desired Joint Values (deg) [8]/1 -> "Select J3, J6"/1
  Rad to Joint Enc/1 -> Demux/1
  Show 1 After At Least 1 Execution Through/1 -> Calibrated/1
  Demux/1 -> HIL Set Encoder Counts/1
  Demux/2 -> HIL Set Encoder Counts/2
  Joint Direction Correction/1 -> 1/Capstan Ratio/1
  "Select J3, J6"/1 -> Joint Direction Correction/1

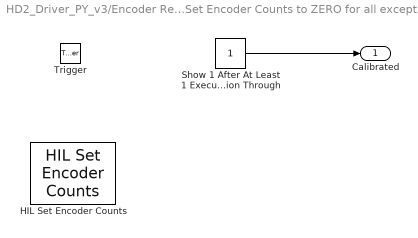
== system HD2_Driver_PY_v3/Encoder Reset (Calibration)/Set Encoder Counts to ZERO for all except Second Joint of 5-bar ==
  Trigger : TriggerPort  VariantControl=Variant
  HIL Set Encoder Counts : quarc_library/Data Acquisition/Generic/Configuration/HIL Set Encoder Counts  object_name=HIL-1  channels=[2 1 5 4 6 7]  source=internal  counts=0  sample_time=-1  active=on  vector_input=off
      settings: AttributesFormatString=(%<object_name>)  SourceProductName=QUARC Targets
  Show 1 After At Least 1 Execution Through : Constant
  Calibrated : Outport  InitialOutput=[0]  VectorParamsAs1DForOutWhenUnconnected=off
  wires:
  Show 1 After At Least 1 Execution Through/1 -> Calibrated/1

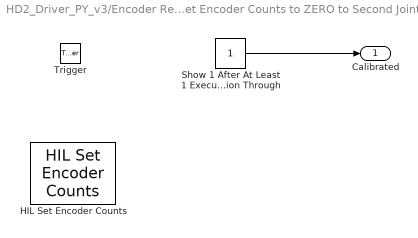
== system HD2_Driver_PY_v3/Encoder Reset (Calibration)/Set Encoder Counts to ZERO to Second Joint of 5-bar ==
  Trigger : TriggerPort  VariantControl=Variant
  HIL Set Encoder Counts : quarc_library/Data Acquisition/Generic/Configuration/HIL Set Encoder Counts  object_name=HIL-1  channels=[0 3]  source=internal  counts=0  sample_time=-1  active=on  vector_input=off
      settings: AttributesFormatString=(%<object_name>)  SourceProductName=QUARC Targets
  Show 1 After At Least 1 Execution Through : Constant
  Calibrated : Outport  InitialOutput=[0]  VectorParamsAs1DForOutWhenUnconnected=off
  wires:
  Show 1 After At Least 1 Execution Through/1 -> Calibrated/1

== matlab function HD2_Driver_PY_v3/Five Bar (PY) - Lower ==
  data: q input; Pos output; LinkLengths input; J output; R output
function [Pos, J, R] = FiveBarKinematics_PY(q, LinkLengths)
%#codegen

% This function computes the kinematics for a 5-Bar Mechanism (POSITIVE Y).

% The 5-Bar has three joints:
% Base Joint (q1): Defined to be rotating about the 5-Bar Native/Inertial x-axis
% First Joint (q2): Defined to be rotating about the local z-axis (when q1=0)
% Second Joint (q3): Also rotating about the local z-axis (when q1=0)
%
% The frames are defined such that when q=[0,0,0], the upper links are
% extending out towards the POSITIVE y direction (of the 5-Bar Native/Inertial frame) 
% while the base offset extends towards the positive x direction, forming a "L" shape.
%
% The LinkLengths contains 3 elements:
%
% L1 = Offset along x-axis of the q2 and q3 from origin
% L2 = Length of the link extending along local y-axis
% L3 = Length of final link from the joint to the end-effecter along local x-axis
%

s1 = sin(q(1));
c1 = cos(q(1));
s2 = sin(q(2));
c2 = cos(q(2));
s3 = sin(q(3));
c3 = cos(q(3));

L1 = LinkLengths(1);
L2 = LinkLengths(2);
L3 = LinkLengths(3);

% Position vector
x = L1 - L2*s2 - L3*s3;
y = L2*c1*c2 + L3*c1*c3;
z = L2*s1*c2 + L3*s1*c3;
Pos = [x, y, z]';

% Jacobian
J11 = 0;
J21 = -L2*s1*c2 - L3*s1*c3;
J31 = L2*c1*c2 + L3*c1*c3;

J12 = -L2*c2;
J22 = -L2*c1*s2;
J32 = -L2*s1*s2;

J13 = -L3*c3;
J23 = -L3*c1*s3;
J33 = -L3*s1*s3;

J = [ J11, J12, J13; J21, J22, J23; J31, J32, J33];

% Unit Base Vector of the end effector frame
% Rotation matrix from base frame (frame 0) to end effector frame (frame e)
% is defined as 
%
% r_0 = R . r_e
%
% where
%
% r_0 = vector expressed in base (5-Bar Native/Inertial) frame
% r_e = vector expressed in end effector frame
% R = [ unitX, unitY, unitZ ]
unitX = [ s3; -c1*c3; -s1*c3];
unitY = [ c3; c1*s3; s1*s3 ];
unitZ = [ 0; -s1; c1 ];
R = [unitX, unitY, unitZ];
